simulink model "Microstick_II_33EP128MC202_Drotek_I2C_MS5611_TempAndPressure"  (Simulink 7.5)
settings: Solver=FixedStepDiscrete  StartTime=0.0  StopTime=10.0  FixedStep=0.01  RelTol=1e-3
undefined symbols (not defined in the file or in its folder): A0, A4, B10, B11, B8, B9, magnitude, Max, ms, P20, P42, P43, Pin, Resol, Slope1, Slope2, us
libraries: simulink x30, MCHP_Blockset x16
(part 1 of 2)
Description:
  | Rapid Prototyping model.
  | Require the MPLAB Blockset for Simulink v3.6 or above. [http://www.microchip.com/SimulinkBlocks]
  | Author: Lubin Kerhuel
  | 
  | Get Temperature (deg) and Pressure (Pa) from MS5611 sensor through I2C bus.
  | Apply compensation based on MS5611 datasheet and EEPROM calibration data.
  | Estimate altitude (m) from the pressure value.
  | 
  | Tested with a Microstick 2 board endowed with a dsPIC 33EP128MC202.
  | The sensor board is the IMU 10DOF V2 from Drotek [http://www.drotek.fr/shop/en/home/62-imu-10dof-mpu6050-hmc5883-ms5611.html].
  | I2C bus is connected to pin B8 (SCL) and B9 (SDA).
  | The Led connected to A0 reflect the MCU load.
settings Model: Creator=Lubin Kerhuel  LastModifiedBy=Lubin Kerhuel
settings OptimizationCC: InlineParams=on  ExpressionDepthLimit=128  OptimizeModelRefInitCode=on  LifeSpan=1
settings DebuggingCC: MultiTaskCondExecSysMsg=warning  FcnCallInpInsideContextMsg=Enable All  StateNameClashWarn=none
settings HardwareCC: ProdBitPerInt=16  ProdIntDivRoundTo=Zero  ProdEndianess=LittleEndian  ProdWordSize=16  ProdHWDeviceType=Generic->Custom
settings ModelReferenceCC: ModelReferenceNumInstancesAllowed=Single
settings RTWCC: SystemTargetFile=MCHP_dsPIC_stf.tlc  TemplateMakefile=MCHP_dsPIC.tmf  Description=Microchip Embedded Target PIC24 dsPIC30 dsPIC33 (real-time)  GenerateReport=on  ProcessScript=MCHP_dsPIC_stf_make_rtw_hook  IncludeHyperlinkInReport=on  LaunchReport=on  GenerateTraceInfo=on  GenerateTraceReport=on  GenerateTraceReportSl=on  GenerateTraceReportSf=on  GenerateTraceReportEml=on
settings CodeAppCC: IgnoreCustomStorageClasses=off  MaxIdLength=255  CustomSymbolStrType=$N$R$M_T
settings STFCustomTargetCC: TargetLibSuffix=_lib.a  IncludeMdlTerminateFcn=off  CombineOutputUpdateFcns=on  SuppressErrorStatus=on  ERTCustomFileBanners=on  SupportContinuousTime=off  SystemTargetFile=MCHP_dsPIC_stf.tlc
settings ERTTargetCC: TargetLibSuffix=_lib.a  MultiwordLength=2048  ParMdlRefBuildCompliant=off  CompOptLevelCompliant=off  IncludeMdlTerminateFcn=off  SuppressErrorStatus=on  ERTFirstTimeCompliant=off  SupportNonInlinedSFcns=on  ModelStepFunctionPrototypeControlCompliant=off  CPPClassGenCompliant=off  InlinedParameterPlacement=NonHierarchical  ERTSrcFileBannerTemplate=MCHP_dsPIC_code_template.cgt  ERTHdrFileBannerTemplate=MCHP_dsPIC_code_template.cgt  ERTDataSrcFileTemplate=MCHP_dsPIC_code_template.cgt  ERTDataHdrFileTemplate=MCHP_dsPIC_code_template.cgt  ERTCustomFileTemplate=MCHP_main.tlc  ConvertIfToSwitch=off
settings CustomProperty: DataType=string  Value=33EP128MC202
settings EnumStrPairs: String=elf

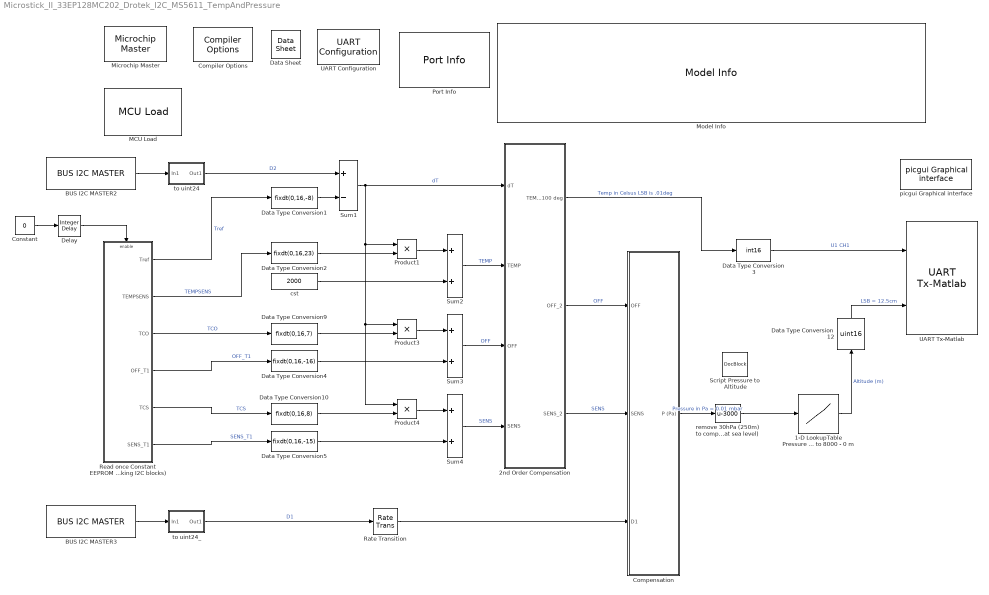
== system Microstick_II_33EP128MC202_Drotek_I2C_MS5611_TempAndPressure ==
  1-D LookupTable Pressure (Pa) to Altitude (m) Validate from 35000 to 101325 Pa  equiv to 8000 - 0 m : Lookup_n-D  NumberOfTableDimensions=1  BreakpointsForDimension1="[  35000  35358  35799  36218  36647  37086  37463  37867  38284  38639  39007  39435  39920  40363  40841  41285  41707  42156  42664  43168  43649  44137  44662  45105  45550  46088  46633  47208  47742  48308  48833  49375  49917  50484  51077  51694  52269  52806  53380  53923  54482  55078  55692  56323  56892  57456  58035  58713  59333  59883  60532  61206  61808  62536  63274  63867  64453  65183  65908  66601  67397  68144  68989  69707  70553  71274  72116  73003  73751  74585  75475  76215  77057  77852  78777  79632  80497  81475  82421  83318  84232  85034  86062  86971  87833  88819  89900  90806  91711  92745  93684  94659  95582  96686  97778  98861  99943  101077  101325]"  BreakpointsForDimension1DataTypeStr=uint32  IndexSearchMethod=Linear search  BeginIndexSearchUsingPreviousIndexResult=on  Table="floor(1e3*[  8.117494150205507  8.047307468888779  7.961635148104636  7.881024806288224  7.799269215467364  7.716406273634682  7.645877610153606  7.570932893861216  7.494252579165659  7.429504315425707  7.362891489741167  7.286054950638820  7.199797399557283  7.121747962190449  7.038306271811481  6.961505205390625  6.889127040412314  6.812766274429189  6.727161471881082  6.643042514664310  6.563500729628082  6.483523422993821  6.398277833852677  6.326975711361185  6.255920317941622  6.170761870543356  6.085312221529850  5.996031117218197  5.913901313824179  5.827657955984869  5.748390298923216  5.667276544272827  5.586880607298991  5.503529360084817  5.417163073045740  5.328158985462957  5.245984553079652  5.169899173342455  5.089261055801668  5.013621668602325  4.936395068204278  4.854760386636663  4.771404863390322  4.686513210163459  4.610620524646503  4.535998870925556  4.460007076468755  4.371798275500042  4.291854427849852  4.221500709507222  4.139153149743339  4.054386808485666  3.979312294958618  3.889311405611741  3.798936060180400  3.726933806801484  3.656311337224353  3.569058183860936  3.483182312323465  3.401808896599658  3.309182745873208  3.223060704013871  3.126556814339318  3.045306345377176  2.950436219991221  2.870307867915639  2.777558779899300  2.680796416665915  2.599934631636417  2.510555168885454  2.416062414745815  2.338179944094234  2.250303556346946  2.168043151867678  2.073183126461139  1.986300471936425  1.899166943670672  1.801559157130934  1.708043624979844  1.620171272121821  1.531418009471097  1.454180476082605  1.356035738721541  1.270039785659123  1.189159990168402  1.097429821079197  0.997804296165603  0.915051309155737  0.833054446807197  0.740167719936515  0.656538791425999  0.570418854500065  0.489551295792444  0.393651965119672  0.299663361166764  0.207285159821775  0.115806970943886  0.020789079348666  0.000124270049324])"  TableDataTypeStr=fixdt(0,16,3)  IntermediateResultsDataTypeStr=fixdt(1,32,18)  ExtrapMethod=None - Clip  UseLastTableValue=on  OutDataTypeStr=fixdt(0,16,3)  RndMeth=Simplest  FractionDataTypeStr=fixdt(1,32,18)  InputSameDT=on
  2nd Order Compensation : Subsystem
  BUS I2C MASTER2 : MCHP_Blockset/BUS I2C/BUS I2C MASTER  I2CRef=1  I2C_IntPriority=5  I2Csequence_txt="Initial-Configuration$     ---     $Start$Write Address:{[0x77]}    % Componnent address$Write Data (x1)  Write:{[0x00]}      % ADC Read$Re-Start$Read Data (x3)  Read:{D2}    % Read D2$Re-Start$Write Data (x1)  Write:{[0x48]}      % Cmd conversion D1 (OSR 4096)$Stop"  I2Csequence_num=[BFF0000000000000 40E0600000000000 412E848000000000 412E9EA0F694FA01]$[4070000000000000]$[3FF0000000000000 40E0200000000000 40F86A0000000000 40F866E066594CA2]$[4040000000000000 0000000000000000 0000000000000000 405DC00000000000]$[4050000000000000 3FF0000000000000 0000000000000000 0000000000000000]$[4008000000000000 40E0200000000000 40F86A0000000000 40F866E066594CA2]$[4060000000000000 4008000000000000]$[4008000000000000 40E0600000000000 40F86A0000000000 40F866E066594CA2]$[4050000000000000 3FF0000000000000 0000000000000000 4052000000000000]$[4000000000000000 40E0600000000000 40F86A0000000000 40F866E066594CA2]  InitialConfigurationNum=0  PIN_SDA_TXT=B9 / Pin[18]  PIN_SCL_TXT=B8 / Pin[17]  S_INPUT="[5  5]"  S_OUTPUT=[5]  S_INPUT_Size="[2  2]"  S_OUTPUT_Size=[4]  BlockingMode=off  SampleTime=[.02 0]  MCHP_MASTERLINK=Microstick_II_33EP128MC202_Drotek_I2C_MS5611_TempAndPressure/Microchip Master  MCHP_PORT={I2C 1 Clock}{SCL1}13:0:B8;{I2C 1 SDA}{SDA1}13:0:B9;  ORDERING=0
  BUS I2C MASTER3 : MCHP_Blockset/BUS I2C/BUS I2C MASTER  I2CRef=1  I2C_IntPriority=5  I2Csequence_txt="Initial-Configuration$     ---     $Start$Write Address:{[0x77]}    % Componnent address$Write Data (x1)  Write:{[0x00]}      % ADC Read$Re-Start$Read Data (x3)  Read:{D1}    % Read D1$Re-Start$Write Data (x1)  Write:{[0x58]}      % Cmd conversion D2 (OSR 4096)$Stop"  I2Csequence_num=[BFF0000000000000 40E0600000000000 412E848000000000 412E9EA0F694FA01]$[4070000000000000]$[3FF0000000000000 40E0200000000000 40F86A0000000000 40F866E066594CA2]$[4040000000000000 0000000000000000 0000000000000000 405DC00000000000]$[4050000000000000 3FF0000000000000 0000000000000000 0000000000000000]$[4008000000000000 40E0200000000000 40F86A0000000000 40F866E066594CA2]$[4060000000000000 4008000000000000]$[4008000000000000 40E0600000000000 40F86A0000000000 40F866E066594CA2]$[4050000000000000 3FF0000000000000 0000000000000000 4056000000000000]$[4000000000000000 40E0600000000000 40F86A0000000000 40F866E066594CA2]  InitialConfigurationNum=0  PIN_SDA_TXT=B9 / Pin[18]  PIN_SCL_TXT=B8 / Pin[17]  S_INPUT="[5  5]"  S_OUTPUT=[5]  S_INPUT_Size="[2  2]"  S_OUTPUT_Size=[4]  BlockingMode=off  SampleTime=[.02 0.01]  MCHP_MASTERLINK=Microstick_II_33EP128MC202_Drotek_I2C_MS5611_TempAndPressure/Microchip Master  MCHP_PORT={I2C 1 Clock}{SCL1}13:0:B8;{I2C 1 SDA}{SDA1}13:0:B9;  ORDERING=0
  Compensation : Subsystem
  Compiler Options : MCHP_Blockset/System Configuration/Compiler Options  Priority=1  LATEST_CMPLR=on  COMP_LIST=Dynamic Options  COMP_LIST_TXT=xc16 - v1.26  USE_64BIT_DOUBLE=off  MCHP_MULTITHREAD_COMPILATION=on  MCHP_MASTERLINK=Microstick_II_33EP128MC202_Drotek_I2C_MS5611_TempAndPressure/Microchip Master  OPTIMIZATION_LEVEL=3  MPLAB_LINKLIB=default  MPLAB_LINKLIB1=default  UNROLL_LOOPS=on  OMIT_FRAME_POINTER=off  PROCEDURAL_ABSTRACTION=off  MCONST=in data memory  MDATA=Use only memory below address 8192 (faster)  MSCALAR=Use only memory below address 8192 (faster)  MCODE=is less than 32768 (faster)  HEAP_SIZE=0  OMF=elf  DEBUG_INFO=off  AssemblyListing=off  ProduceHexOutput=on
  Constant : Constant  Value=0
  Data Sheet : MCHP_Blockset/System Info/Data Sheet  DOC_Type=datasheet  DOC_MCHP_Id=33FJ64MC802  DOC_FileLastCheckTime=[0 0 0 0 0 0]  cpy_MCHP_Id=33EP128MC202  MCHP_MASTERLINK=Microstick_II_33EP128MC202_Drotek_I2C_MS5611_TempAndPressure/Microchip Master
      settings: AttributesFormatString=%<cpy_MCHP_Id>
  Data Type Conversion1 : DataTypeConversion  OutDataTypeMode=Specify via dialog  OutDataType=fixdt(0,16,-8)  OutDataTypeStr=fixdt(0,16,-8)  ConvertRealWorld=Stored Integer (SI)
  Data Type Conversion10 : DataTypeConversion  OutDataTypeMode=Specify via dialog  OutDataType=fixdt(0,16,8)  OutDataTypeStr=fixdt(0,16,8)  ConvertRealWorld=Stored Integer (SI)
  Data Type Conversion12 : DataTypeConversion  OutDataTypeMode=uint16  OutDataTypeStr=uint16  ConvertRealWorld=Stored Integer (SI)
  Data Type Conversion2 : DataTypeConversion  OutDataTypeMode=Specify via dialog  OutDataType=fixdt(0,16,23)  OutDataTypeStr=fixdt(0,16,23)  ConvertRealWorld=Stored Integer (SI)
  Data Type Conversion3 : DataTypeConversion  OutDataTypeMode=int16  OutDataTypeStr=int16
  Data Type Conversion4 : DataTypeConversion  OutDataTypeMode=Specify via dialog  OutDataType=fixdt(0,16,-16)  OutDataTypeStr=fixdt(0,16,-16)  ConvertRealWorld=Stored Integer (SI)
  Data Type Conversion5 : DataTypeConversion  OutDataTypeMode=Specify via dialog  OutDataType=fixdt(0,16,-15)  OutDataTypeStr=fixdt(0,16,-15)  ConvertRealWorld=Stored Integer (SI)
  Data Type Conversion9 : DataTypeConversion  OutDataTypeMode=Specify via dialog  OutDataType=fixdt(0,16,7)  OutDataTypeStr=fixdt(0,16,7)  ConvertRealWorld=Stored Integer (SI)
  Delay : simulink/Discrete/Integer Delay  vinit=1  samptime=-1  NumDelays=1
  MCU Load : MCHP_Blockset/Profiling/MCU Load  MCULoadPin=Dynamic Options  MCULoadPin_TXT=A0 / Pin[2]  MCULoadMeasure=off  TIMER_Resolution=Dynamic Options  TIMER_Resolution_TXT="Resol: 0.1333(us)  -  Max: 8.74(ms)"  MCHP_PORT={MCU Load Pin}{MCU_Load}0:1:A0;  MCHP_TIMER_REQUEST={MCU_Load}{MCU_Load}21:5:0:0:[]:524288;  MCHP_TIMER_RESULT=[2 65535 ]  MCHP_MASTERLINK=Microstick_II_33EP128MC202_Drotek_I2C_MS5611_TempAndPressure/Microchip Master  MCHP_COMPILED_INFO="CompiledSampleTime= [Inf   0 ];CompiledInportDataTypes=[ ];CompiledInportDataWidth=[];"  Info="Timer 2:  Resol: 133.304768(ns)  -  Max: 8.73626(ms)"  SampleTime=-1
  Microchip Master : MCHP_Blockset/System Configuration/Microchip Master  Priority=1  PICREF=33EP128MC202  TIMESTEP_REF="Timer  ( 0.01s + [-9.5218e-005%] ==> 0.01s )"  BUSYFLAG=Dynamic Options  BUSYFLAG_TXT=None  PWRTEN=PWRT enabled  BOREN=Disable  BODENV=2.7V  BORV=Brown-out Reset set at 2.0V  FPWRT=64ms  DSBOREN=Deep Sleep BOR enabled in Deep Sleep  DSLPBOR=Deep Sleep BOR enabled in Deep Sleep  MCLRE=Enabled  SMCLR=MCLR pin generates a normal system Reset  PMDL1WAY=Allow only one reconfiguration  RSTPRI=Device will obtain reset instruction from Primary flash  TEMP=Not used  SOSCSRC=Analog Mode for use with crystal  SOSCSEL=Secondary oscillator configured for high-power operation  IOL1WAY=Allow only one reconfiguration  ALTVREF=Voltage reference input; ADC =RA9/RA10 Comparator =RA9;RA10  DISUVREG=Regulator is disabled  DSSWEN=Deep Sleep is controlled by the register bit DSEN  LPCFG=Disabled - regardless of RETEN  RTCBAT=RTC operation is continued through VBAT  VBTBOR=VBAT BOR enabled  WUTSEL=Default regulator start-up time used  POWERSAVE=off  FNOSC=Internal Fast RC (FRC)  FPR=ECIO w/ PLL 16x  FOSFPR=HS3 w/PLL 16x  FOS=Internal Fast RC  FRANGE=High Range  OSCILLATOR_SELECT=Internal Fast RC (FRC)  OSCILLATOR_SELECT_spd=Internal Fast RC (FRC)  QUARTZ=7.37e+06  QUARTZ_spd=7.37e+06  POSCGAIN=2x gain setting  POSCBOOST=Boost the kick start of the oscillator  SOSCGAIN=2x gain setting  SOSCBOOST=Boost the kick start of the oscillator  ACTIV_PLL=on  ACTIV_PLL_spd=on  MIPS_DESIRED=60e6  MIPS_DESIRED_spd=60e6  FPLLMUL=24x Multiplier  FPLLIDIV=12x Divider  POSCFREQ=Primary oscillator/external clock input frequency greater than 8MHz  POSCMD=XT Crystal Oscillator Mode  POSCMOD=Primary Oscillator Disabled  MIPS=60.012857142857136 * 1e6  FPLLODIV=PLL Divide by 256  PLLKEN=Clock switch to PLL source will wait until the PLL lock signal is valid.  FCKSM=Clock switching is enabled;Fail-safe Clock Monitor is disabled  FCKSMEN=Sw Disabled; Mon Disabled  IESO=Start up with FRC; then switch  DSWDTPS=1:2;147;483;648 (25.7 Days)  FWDTEN=Disable  FWDTWINSZ=Window size is 25%  FWPSA=1:512  FWPSA0=1:128  FWPSB=1:16  WDT=Disable  WDTPOST=1:32768  WDTPRE=1:128  WDTPS=1:32768  WINDIS=Watchdog Timer in Non-Window mode  WWDTEN=Non-Window mode  DSWDTEN=DSWDT enabled  DSWDTOSC=DSWDT uses Low Power RC Oscillator (LPRC)  FPBDIV=Pb_Clk is Sys_Clk/8  FSOSCEN=Enabled  LPRCSEL=High Power; High Accuracy Mode  OSCIOFCN=OSCO/CLKO/RA3 functions as CLKO (FOSC/2)  OSCIOFNC=OSC2 is general purpose digital I/O pin  LVRCFG=Low Voltage regulator is not available  PLL_96MHZ=Enabled  PLL96MHZ=96 MHz PLL Startup is enabled automatically on start-up  PLLDIV=PLL is disabled  WDTCLK=WDT uses LPRC  WDTCMX=WDT clock source is determined by the WDTCLK Configuration bits  WDTWIN=WDT Window is 25% of WDT period  APL=Aux Flash Code protect is disabled  APLK=Aux Flash Write Protection or Code Protection is Enabled  AWRP=Aux Flash may be written  BSS=No boot program Flash segment  BWP=Protection Disabled  BWRP=Boot Segment may be written  CP=Protection Disabled  EBS=No Boot EEPROM  ESS=No Segment Data EEPROM  GCP=General Segment Code protect is disabled  GSS=User program memory is not code-protected  GSS0=No protection  GSSK=General Segment Write Protection or Code Protection is Enabled  GWRP=General Segment may be written  PWP=Disable  RBS=No Boot RAM  RSS=No Secure RAM  SSS=No Secure Segment  SWRP=Secure segment may be written  WPCFG=Disable  WPDIS=Disable  WPEND=Write Protect from WPFP to the last page of memory  WPFP=Page 127 (0x1FC00)  ICESEL=Communicate on PGEC1/PGED1  ICS=Communicate on PGEC1 and PGED1  JTAGEN=Disable  COE=Reset Into Operational Mode  RES=Not used  DEBUG=Debugger is disabled  BACKBUG=Not used  BKBUG=Device resets into Operational mode  ALTI2C=I2C mapped to SDA1/SCL1 pins  ALTI2C1=I2C1 mapped to ASDA1/ASCL1 pins  ALTI2C2=I2C2 mapped to SDA2/SCL2 pins  ALTQIO=QEA1; QEB1; INDX1 are selected as inputs to QEI1  ALTSS1=SS1A is selected as the I/O pin for SPI1  CMPPOL0=Hysteresis is applied to falling edge  CMPPOL1=Hysteresis is applied to falling edge  FCANIO=Default CAN I/O  FETHIO=Default Ethernet I/O  FMIIEN=MII Enabled  FSRSSEL=SRS Priority 7  FUSBIDIO=Controlled by the USB Module  FVBUSONIO=Controlled by USB Module  HPOL=Active High  HYST0=45 mV Hysteresis  HYST1=45 mV Hysteresis  I2C1SEL=Use Default SCL1/SDA1 Pins For I2C1  LPOL=Active High  PWMPIN=Control with PORT/TRIS regs  RTCOSC=RTCC uses Secondary Oscillator (SOSC)  UPLLEN=Disabled and bypassed  UPLLIDIV=12x Divider  ATMOD8=Not used  ALTPMP=EPMP pins are in default location mode  I2C2SEL=I2C2 is multiplexed to SDA2/RA3 and SCL2/RA2  ALTADREF=AVREF+/AVREF- are mapped to RA9/RA10  ALTCVREF=CVREF+/CVREF- are mapped to RA9/RA10  PWMLOCK=PWM registers may be written without key sequence  MCHP_TIMER_REQUEST={Time Step}{TS}0:2:3:1:[]:600128.5714285714;  MCHP_TIMER_RESULT=[1 9376.0089285714239 ]  MCHP_PLLRegisters="[5    226  16387     -1]"  MCHPVAR=MCHP.fcy.periph=MCHP_Fun.Hex2num('[418C9DC9C9249248]');MCHP.fcy.MIPS=MCHP_Fun.Hex2num('[418C9DC9C9249248]');MCHP.PowerSave=0;MCHP.TimeStepFactor=MCHP_Fun.Hex2num('[3FEFFFFE00CDCD2A]');MCHP.TimeStep_Timer=1;MCHP.NTIMERS=5;MCHP.id.name='33EP128MC202';MCHP.id.N=reshape([33 128 202],1,3);MCHP.id.L=reshape({ 'EP','MC',''},1,3);MCHP.id.Arch=3;MCHP.periph.PPS.reg_RPINRx=reshape([-1 1 1 -1 -1 -1 1 -1 -1 -1 -1 -1 -1 -1 1 1 1 1 -1 -1 -1 -1 -1 -1 1 1 -1 -1 1 1 1 1 -1 -1 -1 -1 1 -1 1 -1 -1 -1 -1 -1 1 1 1 -1 -1 -1 -1 -1 1 -1 -1 -1 -1 -1 -1 -1 -1 -1 -1 -1 -1 -1 -1 -1 -1 -1 -1 -1 -1 -1 -1 1 -1 1 1 1],1,80);MCHP.PPS.dsPIC.RP=reshape([-1 -1 -1 -1 -1 -1 -1 -1 -1 -1 -1 -1 -1 -1 -1 -1 -1 -1 -1 -1 4 -1 -1 -1 -1 -1 -1 -1 -1 -1 -1 -1 -1 -1 -1 19 20 21 22 23 24 25 26 27],1,44);MCHP.PPS.dsPIC.RPI=reshape([-1 -1 -1 -1 -1 -1 -1 -1 -1 -1 -1 -1 -1 -1 -1 -1 -1 -1 -1 -1 -1 -1 -1 -1 -1 -1 -1 -1 -1 -1 -1 -1 16 17 18 -1 -1 -1 -1 -1 -1 -1 -1 -1 28 29 30 31],1,48);MCHP.PPS.dsPIC.RPINR_list=reshape({ '1','INT1','INT2','INT3','INT4','T1CK','T2CK','T3CK','T4CK','T5CK','T6CK','T7CK','T8CK','T9CK','IC1','IC2','IC3','IC4','IC5','IC6','IC7','IC8','OCFA','OCFB','FLT1','FLT2','FLT3','FLT4','QEA1','QEB1','INDX1','HOME1','QEA2','QEB2','INDX2','HOME2','U1RX','U1CTS','U2RX','U2CTS','SDI1','SCK1','SS1','44','SDI2','SCK2','SS2','48','CSDIR','CSCK','COFS','52','C1RX','C2RX','U3RX','U3CTS','U4RX','U4CTS','SDI3','SCK3','SS3','62','SDI4','SCK4','SS4','66','IC9','IC10','IC11','IC12','IC13','IC14','IC15','IC16','OCFC','SYNCI1','SYNCI2','DTCMP1','DTCMP2','DTCMP3','DTCMP4','DTCMP5','DTCMP6','DTCMP7','FLT5','FLT6','FLT7','FLT8','89','SENT1','SENT2','92'},1,92);MCHP.PPS.dsPIC.RPOR_list=reshape({ '1','U1TX','U1RTS','U2TX','U2RTS','SDO1','SCK1','SS1','SDO2','SCK2','SS2','CSDO','CSCK','COFS','C1TX','C2TX','OC1','OC2','OC3','OC4','OC5','OC6','OC7','OC8','C1OUT','C2OUT','C3OUT','U3TX','U3RTS','U4TX','U4RTS','SDO3','SCK3','SS3','SDO4','SCK4','SS4','OC9','OC10','OC11','OC12','OC13','OC14','OC15','OC16','SYNCO1','SYNCO2','QEI1CCMP','QEI2CCMP','REFCLK','C4OUT','C5OUT','52','53','54','55','56','SENT1','SENT2'},1,59);MCHP.PPS.map_RPnR_RPORx=reshape([20 35 36 37 38 39 40 41 42 43],1,10);MCHP.Rx=reshape([2 4 -1 -1 -1 -1 -1 -1 -1 -1 -1 3 5 -1 -1 -1 -1 -1 -1 -1 -1 -1 9 6 -1 -1 -1 -1 -1 -1 -1 -1 -1 10 7 -1 -1 -1 -1 -1 -1 -1 -1 -1 12 11 -1 -1 -1 -1 -1 -1 -1 -1 -1 -1 14 -1 -1 -1 -1 -1 -1 -1 -1 -1 -1 15 -1 -1 -1 -1 -1 -1 -1 -1 -1 -1 16 -1 -1 -1 -1 -1 -1 -1 -1 -1 -1 17 -1 -1 -1 -1 -1 -1 -1 -1 -1 -1 18 -1 -1 -1 -1 -1 -1 -1 -1 -1 -1 21 -1 -1 -1 -1 -1 -1 -1 -1 -1 -1 22 -1 -1 -1 -1 -1 -1 -1 -1 -1 -1 23 -1 -1 -1 -1 -1 -1 -1 -1 -1 -1 24 -1 -1 -1 -1 -1 -1 -1 -1 -1 -1 25 -1 -1 -1 -1 -1 -1 -1 -1 -1 -1 26 -1 -1 -1 -1 -1 -1 -1 -1 -1],11,16);MCHP.ADC.ANtype=reshape([3 0],1,2);MCHP.ADC.ADCONx=reshape([47103 59391 40959 263 0 0],1,6);MCHP.ADC.ADCHS_0=reshape([40863 1799],1,2);MCHP.ADC.Flags=reshape([1 0],1,2);MCHP.ADC.Buffer=reshape([16 -1],1,2);MCHP.ADC.port=reshape([0 1 16 17 18 19 -1 -1 -1 -1 -1 -1 -1 -1 -1 -1 -1 -1 -1 -1 -1 -1 -1 -1 -1 -1 -1 -1 -1 -1 -1 -1 -1 -1 -1 -1 -1 -1 -1 -1 -1 -1 -1 -1 -1 -1 -1 -1 -1 -1 -1 -1 -1 -1 -1 -1 -1],1,57);MCHP.ADC.port_VrefP=17;MCHP.ADC.port_VrefM=16;MCHP.ADC.port_AVdd=-1;MCHP.ADC.port_AVss=-1;MCHP.memory.RAM=16384;MCHP.memory.RAM_XBegin=4096;MCHP.memory.RAM_YBegin=12288;MCHP.memory.RAM_dma=reshape([-1 -1],1,2);MCHP.DMA.Num=4;MCHP.DMA.CNTmax=16383;MCHP.QEI.QEICONx=reshape([49023 -1 -1 -1 -1 -1],1,6);MCHP.QEI.QEItype=1;MCHP.QEI.Port_QEI_INDX=reshape([-1 -1],1,2);MCHP.QEI.Port_QEI_QEA=reshape([-1 -1],1,2);MCHP.QEI.Port_QEI_QEB=reshape([-1 -1],1,2);MCHP.QEI.Port_QEI_UPDN=reshape([-1 -1],1,2);MCHP.INT.Port=reshape([23 32767 32767 -1 -1],1,5);MCHP.PWM_HS.Flags=reshape([3 1 0],1,3);MCHP.PWM.port_FLT=reshape([-1 -1 -1 -1 -1 -1 -1 -1 -1 -1 -1 -1 -1 -1 -1 -1 -1 -1 -1 -1 -1 -1 -1 -1 -1 -1 -1 -1 -1 -1 -1 -1 20],1,33);MCHP.PWM.PWMRef=-1;MCHP.PWM.Flag=0;MCHP.PWM.Port_PWM_l=reshape([31 -1 29 -1 27 -1 -1 -1 -1 -1 -1 -1 -1 -1 -1 -1 -1 -1],2,9);MCHP.PWM.Port_PWM_h=reshape([30 -1 28 -1 26 -1 -1 -1 -1 -1 -1 -1 -1 -1 -1 -1 -1 -1],2,9);MCHP.IC.Port=reshape([32767 32767 32767 32767 0 0 0 0 0 0 0 0 0 0 0 0],1,16);MCHP.IC.type=1;MCHP.OC.Port=reshape([32767 32767 32767 32767 0 0 0 0 0 0 0 0 0 0 0 0],1,16);MCHP.OC.type=1;MCHP.CN.Port=reshape([-1 -1 -1 -1 -1 -1 -1 -1 -1 -1 -1 -1 -1 -1 -1 -1 -1 -1 -1 -1 -1 -1 -1 -1 -1 -1 -1 -1 -1 -1 -1 -1 -1 -1 -1 -1 -1 -1 -1 -1 -1 -1 -1 -1 -1 -1 -1 -1 -1 -1 -1 -1 -1 -1 -1 -1 -1 -1 -1 -1 -1 -1 -1 -1 -1 -1 -1 -1 -1 -1 -1 -1 -1 -1 -1 -1 -1 -1 -1 -1 -1 -1 -1 -1 -1],1,85);MCHP.CN.PullUp=reshape([31 65535 0 0 0 0 0 0 0 0 0],1,11);MCHP.CN.type=1;MCHP.CN.Flag_PullDown=1;MCHP.SPI.Refs=reshape([1 2 0 0 0 0],1,6);MCHP.SPI.SPIxCON1=8191;MCHP.SPI.SPIxCON2=57347;MCHP.SPI.Port_SDI=reshape([25 -1 -1 -1 -1 -1],1,6);MCHP.SPI.Port_SDO=reshape([24 -1 -1 -1 -1 -1],1,6);MCHP.SPI.Port_SCK=reshape([23 -1 -1 -1 -1 -1],1,6);MCHP.SPI.Port_SS=reshape([16 -1 -1 -1 -1 -1],1,6);MCHP.I2C.Refs=reshape([1 2 0 0 0],1,5);MCHP.I2C.I2CxCON=49151;MCHP.I2C.NewRegName=1;MCHP.I2C.Port_SDA=reshape([-1 -1 -1 -1 -1],1,5);MCHP.I2C.Port_SCL=reshape([-1 -1 -1 -1 -1],1,5);MCHP.I2C.Port_ASDA=reshape([25 21 -1 -1 -1],1,5);MCHP.I2C.Port_ASCL=reshape([24 22 -1 -1 -1],1,5);MCHP.I2C.Fuse_Port_SCL_SDA=reshape([3 1 4 1 -1 -1 -1 -1 -1 -1],2,5);MCHP.I2C.Fuse_Port_ASCL_ASDA=reshape([3 2 4 2 -1 -1 -1 -1 -1 -1],2,5);MCHP.Comp.Port_CVrefin=-1;MCHP.Comp.Port_CVref=-1;MCHP.Comp.Port_CVref1O=24;MCHP.Comp.Port_CVref2O=4;MCHP.Comp.Port_CxOUT=reshape([32767 32767 32767 32767 -1],1,5);MCHP.Comp.Port_OAxOUT=reshape([17 0 -1 -1 -1],1,5);MCHP.Comp.Port_CxINP=reshape([18 1 -1 -1 -1],1,5);MCHP.Comp.Port_CxINM=reshape([19 -1 -1 -1 16 -1 -1 -1 -1 -1 -1 -1 -1 -1 -1 -1 -1 -1 -1 -1],4,5);MCHP.Comp.nComp=reshape([4 0 0],1,3);MCHP.Comp.OpAmp=3;MCHP.Comp.CVRCON=reshape([17663 0],1,2);MCHP.UART.port_Rx=reshape([32767 32767 -1 -1 -1 -1],1,6);MCHP.UART.port_Tx=reshape([32767 32767 -1 -1 -1 -1],1,6);MCHP.UART.port_ARx=reshape([-1 -1],1,2);MCHP.UART.port_ATx=reshape([-1 -1],1,2);MCHP.UART.port_RTS=reshape([32767 32767 -1 -1 -1 -1],1,6);MCHP.UART.port_CTS=reshape([32767 32767 -1 -1 -1 -1],1,6);MCHP.UART.reg_UxMODE=reshape([48127 48127 -1 -1 -1 -1],1,6);MCHP.UART.reg_UxSTA=reshape([61439 61439 -1 -1 -1 -1],1,6);  MCHP_CRC=2807621  BTMODE=Device is in Single Boot (legacy) mode  RES1=Not used  PLLSS=PLL is fed by the Primary oscillator  RES2=Not used  ALTCMPI=C1INC is on RB13; C2INC is on RB9 and C3INC is on RA0  BOREN1=BOR Enabled [When BOREN=1]  ALTRB6=Append the RP6/ASCL1/PMPD6 functions of RB6 to RA1 pin functions  RETCFG=Retention regulator is not available  DFMCY=Not used  BSS2=No Boot Segment  BSEN=No Boot Segment  CWRP=Configuration Segment may be written  CSS=No Protection (other than CWRP)  AIVTDIS=Disable Alternate Vector Table  BSLIM=Not used  WDTEN=Disable  BTSWP=Not used  DBCC=Not used  CTXT1=Not Assigned  CTXT2=Not Assigned  SEQNUM=Not used  nSEQNUM=Not used  BOREN0=Enabled  DMTIVT=Not used  DMTCNT=2^31 (2147483648)  DMTEN=Dead Man Timer is Enabled and cannot be disabled by software  ON=Not used  USERID=Not used  RESERVED1=Not used  PGL1WAY=Allow only one reconfiguration  FPLLRNG=34-68 MHz Input  FPLLICLK=FRC is input to the System PLL  FPLLMULT=PLL Multiply by 128  UPLLFSEL=USB PLL input is 24 MHz  DMTINTV=Window/Interval value is 127/128 counter value  WDTSPGM=WDT stops during Flash programming  FDMTEN=Deadman Timer is disabled  TRCEN=Trace features in the CPU are enabled  BOOTISA=Boot code and Exception code is MIPS32  FECCCON=ECC and Dynamic ECC are disabled (ECCCON bits are writable)  EXTDDRSIZE=External DDR2 Size is 128 MB  FSLEEP=Flash is powered down when the device is in Sleep mode  DBGPER=Allow CPU access to all permission regions  EJTAGBEN=Normal EJTAG functionality  TSEQ=Not used  CSEQ=Not used
  Model Info : simulink/Model-Wide Utilities/Model Info  SystemSampleTime=-1  InitialBlockCM=none  BlockCM=none  Frame=off  DisplayStringWithTags=%<Description>  HorizontalTextAlignment=Center  LeftAlignmentValue=0.5  SourceBlockDiagram=Microstick_II_33EP128MC202_Drotek_I2C_MS5611_TempAndPressure  TagMaxNumber=20
  Port Info : MCHP_Blockset/System Info/Port Info  MCHP_MASTERLINK=Microstick_II_33EP128MC202_Drotek_I2C_MS5611_TempAndPressure/Microchip Master
  Product1 : Product
  Product3 : Product
  Product4 : Product
  Rate Transition : RateTransition  Integrity=off  Deterministic=off
  Read once Constant EEPROM Calibration data From MS5611 (Blocking I2C blocks) : Subsystem
  Script Pressure to Altitude : simulink/Model-Wide Utilities/DocBlock  SystemSampleTime=-1  DocumentType=Text
      content=|
      | %% The script to compute the lookup table to translate pressure from Pascal unit (Pa) to meters (m) here after
      |
      | func = '44331.5-4946.62*x.^0.190263';   % Model from Pressure (Pa) to altitude (m)
      |
      | xmin = 35000;  xmax = 101325; % Min and max pressure
      | xdt = ufix(32); xscale = 1; % x scaling
      |
      | ydt = ufix(16);
      | yscale = 2^-3;  % y output is altitude, in m. Max value is 8000 thus 13 bits are required for integer part and 3 can be used as fractional part.
      | % y LSB is 12.5 cm
      |
      | rndmeth = 'Floor';
      | errmax = [.2];
      | nptsmax = 256;
      | %spacing = 'even';
      |
      | % Compute lookup table (might take few seconds to compute)
      | [xdata,ydata,errworst] = fixpt_look1_func_approx(func,xmin,xmax,xdt,xscale,ydt,yscale,rndmeth,errmax,nptsmax);
      | % Check results
      | fixpt_look1_func_plot(xdata,ydata,func,xmin,xmax,xdt,xscale,ydt,yscale,rndmeth);
  Sum1 : Sum  Inputs=+-  AccumDataTypeStr=fixdt(1,24,0)  OutDataTypeStr=Inherit: Same as accumulator
  Sum2 : Sum  OutMin=-4000  OutMax=8500  OutDataTypeMode=Specify via dialog  OutDataType=fixdt(1,32,17)  OutDataTypeStr=fixdt(1,32,17)
  Sum3 : Sum  OutMin=-8589672450  OutMax=12884705280  OutDataTypeMode=Specify via dialog  OutDataType=fixdt(1,41,6)  OutDataTypeStr=fixdt(1,41,6)
  Sum4 : Sum  OutMin=-4294836225  OutMax=6442352640  OutDataTypeMode=Specify via dialog  OutDataType=fixdt(1,41,7)  OutDataTypeStr=fixdt(1,41,7)
  UART Configuration : MCHP_Blockset/BUS UART/UART Configuration  UART_REF=1  BAUD_Choice=Dynamic Options  BAUD_Choice_TXT="115200         [+0.18%]"  BAUD_Choice_IR=Dynamic Options  BAUD_Choice_IR_TXT=[]  BAUD_Custom=115200  IRDA=off  ALT_IO=on  PIN_RX=Dynamic Options  PIN_RX_TXT=B11 / P43 / Pin[22]  PIN_TX=Dynamic Options  PIN_TX_TXT=B10 / P42 / Pin[21]  FlowControl=None  PIN_CTS=Dynamic Options  PIN_CTS_TXT=A4 / P20 / Pin[12]  PIN_RTS=Dynamic Options  PIN_RTS_TXT=A4 / P20 / Pin[12]  MCHP_PORT="{UART1  Tx}{U1TX}3:1:P42;"  MCHP_MASTERLINK=Microstick_II_33EP128MC202_Drotek_I2C_MS5611_TempAndPressure/Microchip Master  MCHP_COM_ExtPil=off  TX_IMPLEMENTATION=Circular Buffer  TX_INT_PRIORITY=5  TX_INT_WHEN=is empty & last char is sent  TX_CIRCULAR_SIZE=32  TX_DMA_CHANNEL="0   (Lowest Priority)"  TX_DMA_SIZE=[]  RX_IMPLEMENTATION=Do not implement Rx  RX_INT_PRIORITY=1  RX_INT_WHEN=receive 1 character  RX_CIRCULAR_SIZE=32  InitSequence_chkbox=off  BAUD_Choice_InitSeq=Dynamic Options  BAUD_Choice_InitSeq_TXT=0  BAUD_Choice_IR_InitSeq=Dynamic Options  BAUD_Choice_IR_InitSeq_TXT=0  BAUD_Custom_InitSeq=0  InitSequence='Hello World'
  UART Tx-Matlab : MCHP_Blockset/BUS UART/UART Tx-Matlab  UART_REF=1  CHANNELS=[1:2]  AllOrNothing=off  SampleTime=-1  MCHP_MASTERLINK=Microstick_II_33EP128MC202_Drotek_I2C_MS5611_TempAndPressure/Microchip Master  MCHP_COMPILED_INFO="CompiledSampleTime= [0.02   0 ];CompiledInportDataTypes=[  4   5 ];CompiledInportDataWidth=[1  1];"
  cst : Constant  Value=2000  OutDataTypeMode=uint16  OutDataTypeStr=uint16
  picgui Graphical interface : MCHP_Blockset/BUS UART/picgui Graphical interface  Nothing=0
  remove 30hPa (250m) to compensate for bad weather forecast (avoir neg value at sea level) : Bias  Bias=-3000
  to uint24 : Subsystem
  to uint24_ : Subsystem
  wires:
  BUS I2C MASTER2/1 -> to uint24/1(In1)
  to uint24/1(Out1) -> Sum1/1  "D2"
  Data Type Conversion1/1 -> Sum1/2
  Sum1/1 -> Product3/1, Product4/1, Product1/1, 2nd Order Compensation/1(dT)  "dT"
  Product1/1 -> Sum2/1
  Data Type Conversion2/1 -> Product1/2
  Product3/1 -> Sum3/1
  Data Type Conversion4/1 -> Sum3/2
  Product4/1 -> Sum4/1
  Data Type Conversion5/1 -> Sum4/2
  Data Type Conversion9/1 -> Product3/2
  Data Type Conversion10/1 -> Product4/2
  Delay/1 -> Read once Constant EEPROM Calibration data From MS5611 (Blocking I2C blocks)/Enable
  Constant/1 -> Delay/1
  cst/1 -> Sum2/2
  Sum2/1 -> 2nd Order Compensation/2(TEMP)  "TEMP"
  Sum3/1 -> 2nd Order Compensation/3(OFF)  "OFF"
  Sum4/1 -> 2nd Order Compensation/4(SENS)  "SENS"
  to uint24_/1(Out1) -> Rate Transition/1  "D1"
  2nd Order Compensation/3(SENS_2) -> Compensation/2(SENS)  "SENS"
  2nd Order Compensation/2(OFF_2) -> Compensation/1(OFF)  "OFF"
  Rate Transition/1 -> Compensation/3(D1)
  BUS I2C MASTER3/1 -> to uint24_/1(In1)
  Read once Constant EEPROM Calibration data From MS5611 (Blocking I2C blocks)/1(Tref) -> Data Type Conversion1/1  "Tref"
  Read once Constant EEPROM Calibration data From MS5611 (Blocking I2C blocks)/2(TEMPSENS) -> Data Type Conversion2/1  "TEMPSENS"
  Read once Constant EEPROM Calibration data From MS5611 (Blocking I2C blocks)/3(TCO) -> Data Type Conversion9/1  "TCO"
  Read once Constant EEPROM Calibration data From MS5611 (Blocking I2C blocks)/4(OFF_T1) -> Data Type Conversion4/1  "OFF_T1"
  Read once Constant EEPROM Calibration data From MS5611 (Blocking I2C blocks)/5(TCS) -> Data Type Conversion10/1  "TCS"
  Read once Constant EEPROM Calibration data From MS5611 (Blocking I2C blocks)/6(SENS_T1) -> Data Type Conversion5/1  "SENS_T1"
  2nd Order Compensation/1(TEMP 1/100 deg) -> Data Type Conversion3/1  "Temp in Celsus LSB is .01deg"
  Data Type Conversion3/1 -> UART Tx-Matlab/1  "U1 CH1"
  Compensation/1(P (Pa)) -> remove 30hPa (250m) to compensate for bad weather forecast (avoir neg value at sea level)/1  "Pressure in Pa = 0.01 mbar"
  remove 30hPa (250m) to compensate for bad weather forecast (avoir neg value at sea level)/1 -> 1-D LookupTable Pressure (Pa) to Altitude (m) Validate from 35000 to 101325 Pa  equiv to 8000 - 0 m/1
  1-D LookupTable Pressure (Pa) to Altitude (m) Validate from 35000 to 101325 Pa  equiv to 8000 - 0 m/1 -> Data Type Conversion12/1  "Altitude (m)"
  Data Type Conversion12/1 -> UART Tx-Matlab/2  "LSB = 12.5cm"

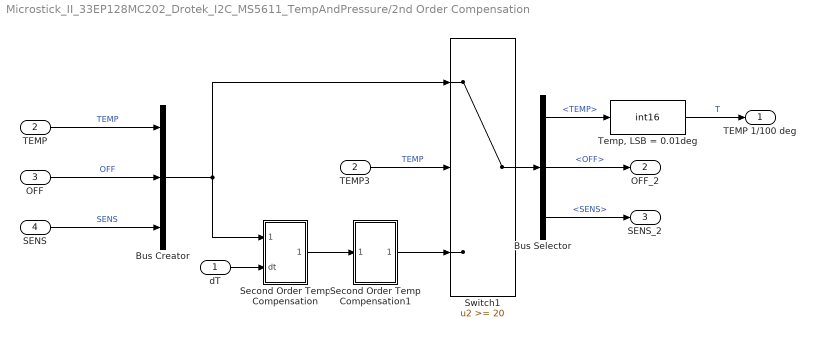
== system Microstick_II_33EP128MC202_Drotek_I2C_MS5611_TempAndPressure/2nd Order Compensation ==
  dT : Inport
  TEMP : Inport  Port=2
  OFF : Inport  Port=3
  SENS : Inport  Port=4
  Bus Creator : BusCreator  Inputs=3
  Bus Selector : BusSelector  OutputSignals=TEMP,OFF,SENS
  Second Order Temp Compensation : Subsystem
  Second Order Temp Compensation1 : Subsystem
  Switch1 : Switch  Threshold=20  InputSameDT=on
  TEMP3 : InportShadow  Port=2
  "Temp, LSB = 0.01deg" : DataTypeConversion  OutDataTypeMode=int16  OutDataTypeStr=int16
  TEMP 1/100 deg : Outport
  OFF_2 : Outport  Port=2
  SENS_2 : Outport  Port=3
  wires:
  TEMP3/1 -> Switch1/2  "TEMP"
  Switch1/1 -> Bus Selector/1
  TEMP/1 -> Bus Creator/1  "TEMP"
  OFF/1 -> Bus Creator/2  "OFF"
  SENS/1 -> Bus Creator/3  "SENS"
  Bus Creator/1 -> Switch1/1, Second Order Temp Compensation/1(In3)
  Second Order Temp Compensation/1(Out1) -> Second Order Temp Compensation1/1(In3)
  Second Order Temp Compensation1/1(Out1) -> Switch1/3
  Bus Selector/1 -> "Temp, LSB = 0.01deg"/1  "<TEMP>"
  Bus Selector/2 -> OFF_2/1  "<OFF>"
  Bus Selector/3 -> SENS_2/1  "<SENS>"
  dT/1 -> Second Order Temp Compensation/2(dt)
  "Temp, LSB = 0.01deg"/1 -> TEMP 1/100 deg/1  "T"

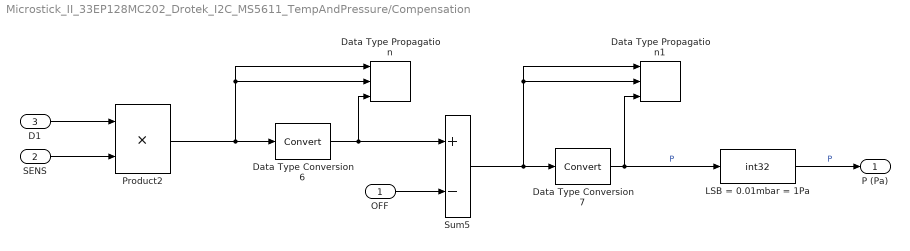
== system Microstick_II_33EP128MC202_Drotek_I2C_MS5611_TempAndPressure/Compensation ==
  OFF : Inport
  SENS : Inport  Port=2
  D1 : Inport  Port=3
  Data Type Propagation : simulink/Signal Attributes/Data Type Propagation  PropDataType=fixdt(1, 16)  IfRefDouble=double  IfRefSingle=single  IsSigned=IsSigned1 or IsSigned2  NumBitsBase=NumBits1  NumBitsMult=1  NumBitsAdd=0  NumBitsAllowFinal=1:128  PropScaling=2^-10  ValuesUsedBestPrec=[5 -7]  SlopeBase=min([Slope1 Slope2])  SlopeMult=2^-21  SlopeAdd=0  BiasBase=Bias1  BiasMult=1  BiasAdd=0
  Data Type Propagation1 : simulink/Signal Attributes/Data Type Propagation  PropDataType=fixdt(1, 16)  IfRefDouble=double  IfRefSingle=single  IsSigned=IsSigned1 or IsSigned2  NumBitsBase=NumBits1  NumBitsMult=1  NumBitsAdd=0  NumBitsAllowFinal=1:128  PropScaling=2^-10  ValuesUsedBestPrec=[5 -7]  SlopeBase=min([Slope1 Slope2])  SlopeMult=2^-15  SlopeAdd=0  BiasBase=Bias1  BiasMult=1  BiasAdd=0
  Data Type Conversion6 : DataTypeConversion  ConvertRealWorld=Stored Integer (SI)
  Data Type Conversion7 : DataTypeConversion  ConvertRealWorld=Stored Integer (SI)
  LSB = 0.01mbar = 1Pa : DataTypeConversion  OutDataTypeMode=int32  OutDataTypeStr=int32
  Product2 : Product  OutMin=-4294836225*(2^24-1)  OutMax=6442352640*(2^24-1)  OutDataTypeMode=Specify via dialog  OutDataType=fixdt(1,64,6)  OutDataTypeStr=fixdt(1,64,6)
  Sum5 : Sum  Inputs=+-  OutDataTypeStr=Inherit: Same as accumulator
  P (Pa) : Outport
  wires:
  Data Type Conversion7/1 -> LSB = 0.01mbar = 1Pa/1, Data Type Propagation1/3  "P"
  D1/1 -> Product2/1
  SENS/1 -> Product2/2
  Product2/1 -> Data Type Propagation/1, Data Type Propagation/2, Data Type Conversion6/1
  Data Type Conversion6/1 -> Data Type Propagation/3, Sum5/1
  OFF/1 -> Sum5/2
  Sum5/1 -> Data Type Propagation1/2, Data Type Propagation1/1, Data Type Conversion7/1
  LSB = 0.01mbar = 1Pa/1 -> P (Pa)/1  "P"

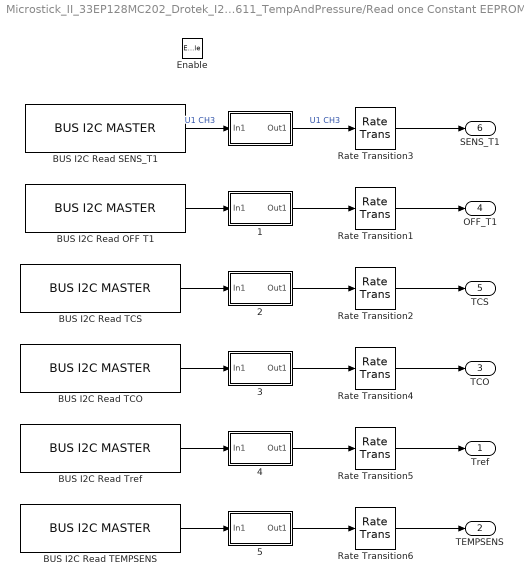
== system Microstick_II_33EP128MC202_Drotek_I2C_MS5611_TempAndPressure/Read once Constant EEPROM Calibration data From MS5611 (Blocking I2C blocks) ==
  Enable : EnablePort
  " " : Subsystem
  " 1" : Subsystem
  " 2" : Subsystem
  " 3" : Subsystem
  " 4" : Subsystem
  " 5" : Subsystem
  BUS I2C Read OFF T1 : MCHP_Blockset/BUS I2C/BUS I2C MASTER  I2CRef=1  I2C_IntPriority=5  I2Csequence_txt="Initial-Configuration$     ---     $Start$Write Address:{[0x77]}    % Componnent address$Write Data (x1)  Write:{[0xA4]}      % PROM Read$Re-Start$Read Data (x2)  Read:{OFF_T1}    % Read OFF_T1$Stop"  I2Csequence_num=[BFF0000000000000 40E0600000000000 412E848000000000 412E9EA0F694FA01]$[4070000000000000]$[3FF0000000000000 40E0200000000000 40F86A0000000000 40F866E066594CA2]$[4040000000000000 0000000000000000 0000000000000000 405DC00000000000]$[4050000000000000 3FF0000000000000 0000000000000000 4064800000000000]$[4008000000000000 40E0200000000000 40F86A0000000000 40F866E066594CA2]$[4060000000000000 4000000000000000]$[4000000000000000 40E0600000000000 40F86A0000000000 410065D9C7810E65]  InitialConfigurationNum=0  PIN_SDA_TXT=B9 / Pin[18]  PIN_SCL_TXT=B8 / Pin[17]  S_INPUT="[5  5]"  S_OUTPUT=[5]  S_INPUT_Size="[2  2]"  S_OUTPUT_Size=[4]  BlockingMode=on  SampleTime=-1  MCHP_MASTERLINK=Microstick_II_33EP128MC202_Drotek_I2C_MS5611_TempAndPressure/Microchip Master  MCHP_PORT={I2C 1 Clock}{SCL1}13:0:B8;{I2C 1 SDA}{SDA1}13:0:B9;  ORDERING=0
  BUS I2C Read SENS_T1 : MCHP_Blockset/BUS I2C/BUS I2C MASTER  I2CRef=1  I2C_IntPriority=5  I2Csequence_txt="Initial-Configuration$     ---     $Start$Write Address:{[0x77]}    % Componnent address$Write Data (x1)  Write:{[0xA2]}      % PROM Read$Re-Start$Read Data (x2)  Read:{SENS_T1}    % Read SENS_T1$Stop"  I2Csequence_num=[BFF0000000000000 40E0600000000000 412E848000000000 412E9EA0F694FA01]$[4070000000000000]$[3FF0000000000000 40E0200000000000 40F86A0000000000 40F866E066594CA2]$[4040000000000000 0000000000000000 0000000000000000 405DC00000000000]$[4050000000000000 3FF0000000000000 0000000000000000 4064400000000000]$[4008000000000000 40E0200000000000 40F86A0000000000 40F866E066594CA2]$[4060000000000000 4000000000000000]$[4000000000000000 40E0600000000000 40F86A0000000000 410065D9C7810E65]  InitialConfigurationNum=0  PIN_SDA_TXT=B9 / Pin[18]  PIN_SCL_TXT=B8 / Pin[17]  S_INPUT="[5  5]"  S_OUTPUT=[5]  S_INPUT_Size="[2  2]"  S_OUTPUT_Size=[4]  BlockingMode=on  SampleTime=-1  MCHP_MASTERLINK=Microstick_II_33EP128MC202_Drotek_I2C_MS5611_TempAndPressure/Microchip Master  MCHP_PORT={I2C 1 Clock}{SCL1}13:0:B8;{I2C 1 SDA}{SDA1}13:0:B9;  ORDERING=0
  BUS I2C Read TCO : MCHP_Blockset/BUS I2C/BUS I2C MASTER  I2CRef=1  I2C_IntPriority=5  I2Csequence_txt="Initial-Configuration$     ---     $Start$Write Address:{[0x77]}    % Componnent address$Write Data (x1)  Write:{[0xA8]}      % PROM Read$Re-Start$Read Data (x2)  Read:{TCO}    % Read TCO$Stop"  I2Csequence_num=[BFF0000000000000 40E0600000000000 412E848000000000 412E9EA0F694FA01]$[4070000000000000]$[3FF0000000000000 40E0200000000000 40F86A0000000000 40F866E066594CA2]$[4040000000000000 0000000000000000 0000000000000000 405DC00000000000]$[4050000000000000 3FF0000000000000 0000000000000000 4065000000000000]$[4008000000000000 40E0200000000000 40F86A0000000000 40F866E066594CA2]$[4060000000000000 4000000000000000]$[4000000000000000 40E0600000000000 40F86A0000000000 410065D9C7810E65]  InitialConfigurationNum=0  PIN_SDA_TXT=B9 / Pin[18]  PIN_SCL_TXT=B8 / Pin[17]  S_INPUT="[5  5]"  S_OUTPUT=[5]  S_INPUT_Size="[2  2]"  S_OUTPUT_Size=[4]  BlockingMode=on  SampleTime=-1  MCHP_MASTERLINK=Microstick_II_33EP128MC202_Drotek_I2C_MS5611_TempAndPressure/Microchip Master  MCHP_PORT={I2C 1 Clock}{SCL1}13:0:B8;{I2C 1 SDA}{SDA1}13:0:B9;  ORDERING=0
  BUS I2C Read TCS : MCHP_Blockset/BUS I2C/BUS I2C MASTER  I2CRef=1  I2C_IntPriority=5  I2Csequence_txt="Initial-Configuration$     ---     $Start$Write Address:{[0x77]}    % Componnent address$Write Data (x1)  Write:{[0xA6]}      % PROM Read$Re-Start$Read Data (x2)  Read:{TCS}    % Read TCS$Stop"  I2Csequence_num=[BFF0000000000000 40E0600000000000 412E848000000000 412E9EA0F694FA01]$[4070000000000000]$[3FF0000000000000 40E0200000000000 40F86A0000000000 40F866E066594CA2]$[4040000000000000 0000000000000000 0000000000000000 405DC00000000000]$[4050000000000000 3FF0000000000000 0000000000000000 4064C00000000000]$[4008000000000000 40E0200000000000 40F86A0000000000 40F866E066594CA2]$[4060000000000000 4000000000000000]$[4000000000000000 40E0600000000000 40F86A0000000000 410065D9C7810E65]  InitialConfigurationNum=0  PIN_SDA_TXT=B9 / Pin[18]  PIN_SCL_TXT=B8 / Pin[17]  S_INPUT="[5  5]"  S_OUTPUT=[5]  S_INPUT_Size="[2  2]"  S_OUTPUT_Size=[4]  BlockingMode=on  SampleTime=-1  MCHP_MASTERLINK=Microstick_II_33EP128MC202_Drotek_I2C_MS5611_TempAndPressure/Microchip Master  MCHP_PORT={I2C 1 Clock}{SCL1}13:0:B8;{I2C 1 SDA}{SDA1}13:0:B9;  ORDERING=0
  BUS I2C Read TEMPSENS : MCHP_Blockset/BUS I2C/BUS I2C MASTER  I2CRef=1  I2C_IntPriority=5  I2Csequence_txt="Initial-Configuration$     ---     $Start$Write Address:{[0x77]}    % Componnent address$Write Data (x1)  Write:{[0xAC]}      % PROM Read$Re-Start$Read Data (x2)  Read:{TEMPSENS}    % Read TEMPSENS$Stop"  I2Csequence_num=[BFF0000000000000 40E0600000000000 412E848000000000 412E9EA0F694FA01]$[4070000000000000]$[3FF0000000000000 40E0200000000000 40F86A0000000000 40F866E066594CA2]$[4040000000000000 0000000000000000 0000000000000000 405DC00000000000]$[4050000000000000 3FF0000000000000 0000000000000000 4065800000000000]$[4008000000000000 40E0200000000000 40F86A0000000000 40F866E066594CA2]$[4060000000000000 4000000000000000]$[4000000000000000 40E0600000000000 40F86A0000000000 410065D9C7810E65]  InitialConfigurationNum=0  PIN_SDA_TXT=B9 / Pin[18]  PIN_SCL_TXT=B8 / Pin[17]  S_INPUT="[5  5]"  S_OUTPUT=[5]  S_INPUT_Size="[2  2]"  S_OUTPUT_Size=[4]  BlockingMode=on  SampleTime=-1  MCHP_MASTERLINK=Microstick_II_33EP128MC202_Drotek_I2C_MS5611_TempAndPressure/Microchip Master  MCHP_PORT={I2C 1 Clock}{SCL1}13:0:B8;{I2C 1 SDA}{SDA1}13:0:B9;  ORDERING=0
  BUS I2C Read Tref : MCHP_Blockset/BUS I2C/BUS I2C MASTER  I2CRef=1  I2C_IntPriority=5  I2Csequence_txt="Initial-Configuration$     ---     $Start$Write Address:{[0x77]}    % Componnent address$Write Data (x1)  Write:{[0xAA]}      % PROM Read$Re-Start$Read Data (x2)  Read:{Tref}    % Read Tref$Stop"  I2Csequence_num=[BFF0000000000000 40E0600000000000 412E848000000000 412E9EA0F694FA01]$[4070000000000000]$[3FF0000000000000 40E0200000000000 40F86A0000000000 40F866E066594CA2]$[4040000000000000 0000000000000000 0000000000000000 405DC00000000000]$[4050000000000000 3FF0000000000000 0000000000000000 4065400000000000]$[4008000000000000 40E0200000000000 40F86A0000000000 40F866E066594CA2]$[4060000000000000 4000000000000000]$[4000000000000000 40E0600000000000 40F86A0000000000 410065D9C7810E65]  InitialConfigurationNum=0  PIN_SDA_TXT=B9 / Pin[18]  PIN_SCL_TXT=B8 / Pin[17]  S_INPUT="[5  5]"  S_OUTPUT=[5]  S_INPUT_Size="[2  2]"  S_OUTPUT_Size=[4]  BlockingMode=on  SampleTime=-1  MCHP_MASTERLINK=Microstick_II_33EP128MC202_Drotek_I2C_MS5611_TempAndPressure/Microchip Master  MCHP_PORT={I2C 1 Clock}{SCL1}13:0:B8;{I2C 1 SDA}{SDA1}13:0:B9;  ORDERING=0
  Rate Transition{1..6} (6 alike) : RateTransition  Integrity=off  Deterministic=off
  Tref : Outport
  TEMPSENS : Outport  Port=2
  TCO : Outport  Port=3
  OFF_T1 : Outport  Port=4
  TCS : Outport  Port=5
  SENS_T1 : Outport  Port=6
  wires:
  BUS I2C Read TCO/1 -> " 3"/1(In1)
  BUS I2C Read Tref/1 -> " 4"/1(In1)
  " "/1(Out1) -> Rate Transition3/1  "U1 CH3"
  Rate Transition3/1 -> SENS_T1/1
  BUS I2C Read TCS/1 -> " 2"/1(In1)
  BUS I2C Read OFF T1/1 -> " 1"/1(In1)
  BUS I2C Read TEMPSENS/1 -> " 5"/1(In1)
  BUS I2C Read SENS_T1/1 -> " "/1(In1)  "U1 CH3"
  " 1"/1(Out1) -> Rate Transition1/1
  " 2"/1(Out1) -> Rate Transition2/1
  " 3"/1(Out1) -> Rate Transition4/1
  " 4"/1(Out1) -> Rate Transition5/1
  " 5"/1(Out1) -> Rate Transition6/1
  Rate Transition1/1 -> OFF_T1/1
  Rate Transition2/1 -> TCS/1
  Rate Transition4/1 -> TCO/1
  Rate Transition6/1 -> TEMPSENS/1
  Rate Transition5/1 -> Tref/1

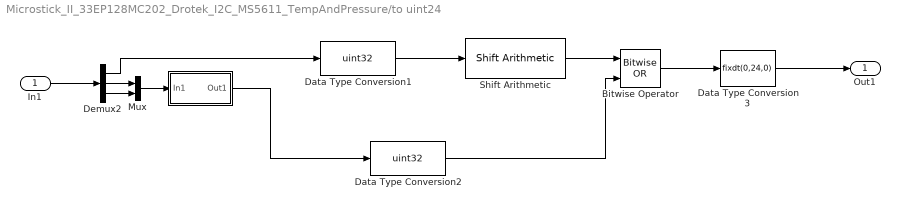
== system Microstick_II_33EP128MC202_Drotek_I2C_MS5611_TempAndPressure/to uint24 ==
  In1 : Inport
  " " : Subsystem
  Bitwise Operator : simulink/Logic and Bit Operations/Bitwise Operator  logicop=OR  UseBitMask=off  NumInputPorts=2  BitMask=bin2dec('11011001')  BitMaskRealWorld=Stored Integer
  Data Type Conversion1 : DataTypeConversion  OutDataTypeMode=uint32  OutDataTypeStr=uint32
  Data Type Conversion2 : DataTypeConversion  OutDataTypeMode=uint32  OutDataTypeStr=uint32
  Data Type Conversion3 : DataTypeConversion  OutDataTypeMode=Specify via dialog  OutDataType=fixdt(0,24,0)  OutDataTypeStr=fixdt(0,24,0)  ConvertRealWorld=Stored Integer (SI)
  Demux2 : Demux  Outputs=3
  Mux : Mux  Inputs=2
  Shift Arithmetic : simulink/Logic and Bit Operations/Shift Arithmetic  SystemSampleTime=-1  nBitShiftRight=-16  nBinPtShiftRight=0
  Out1 : Outport
  wires:
  In1/1 -> Demux2/1
  Shift Arithmetic/1 -> Bitwise Operator/1
  Demux2/1 -> Data Type Conversion1/1
  Mux/1 -> " "/1(In1)
  Demux2/2 -> Mux/1
  Bitwise Operator/1 -> Data Type Conversion3/1
  Demux2/3 -> Mux/2
  " "/1(Out1) -> Data Type Conversion2/1
  Data Type Conversion2/1 -> Bitwise Operator/2
  Data Type Conversion1/1 -> Shift Arithmetic/1
  Data Type Conversion3/1 -> Out1/1

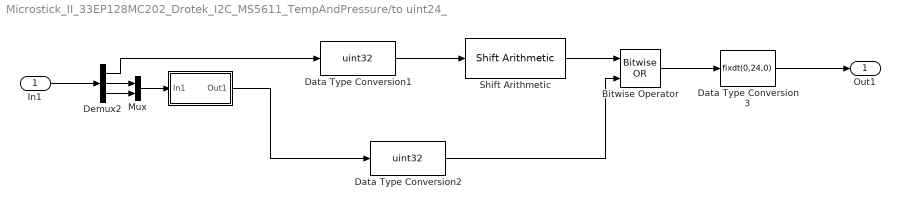
== system Microstick_II_33EP128MC202_Drotek_I2C_MS5611_TempAndPressure/to uint24_ ==
  In1 : Inport
  " " : Subsystem
  Bitwise Operator : simulink/Logic and Bit Operations/Bitwise Operator  logicop=OR  UseBitMask=off  NumInputPorts=2  BitMask=bin2dec('11011001')  BitMaskRealWorld=Stored Integer
  Data Type Conversion1 : DataTypeConversion  OutDataTypeMode=uint32  OutDataTypeStr=uint32
  Data Type Conversion2 : DataTypeConversion  OutDataTypeMode=uint32  OutDataTypeStr=uint32
  Data Type Conversion3 : DataTypeConversion  OutDataTypeMode=Specify via dialog  OutDataType=fixdt(0,24,0)  OutDataTypeStr=fixdt(0,24,0)  ConvertRealWorld=Stored Integer (SI)
  Demux2 : Demux  Outputs=3
  Mux : Mux  Inputs=2
  Shift Arithmetic : simulink/Logic and Bit Operations/Shift Arithmetic  SystemSampleTime=-1  nBitShiftRight=-16  nBinPtShiftRight=0
  Out1 : Outport
  wires:
  Data Type Conversion3/1 -> Out1/1
  Data Type Conversion1/1 -> Shift Arithmetic/1
  Data Type Conversion2/1 -> Bitwise Operator/2
  " "/1(Out1) -> Data Type Conversion2/1
  Demux2/3 -> Mux/2
  Bitwise Operator/1 -> Data Type Conversion3/1
  Demux2/2 -> Mux/1
  Mux/1 -> " "/1(In1)
  Demux2/1 -> Data Type Conversion1/1
  Shift Arithmetic/1 -> Bitwise Operator/1
  In1/1 -> Demux2/1

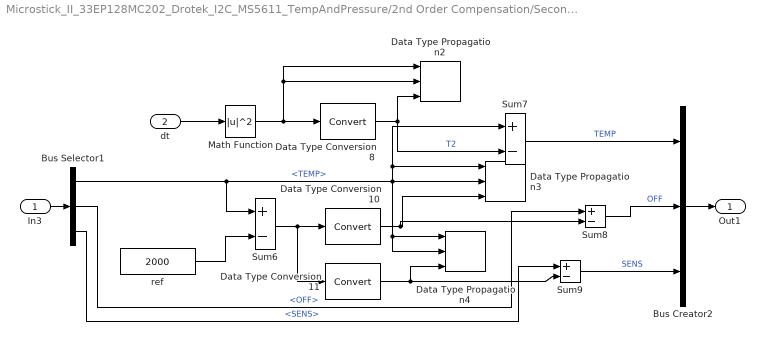
== system Microstick_II_33EP128MC202_Drotek_I2C_MS5611_TempAndPressure/2nd Order Compensation/Second Order Temp Compensation ==
  In3 : Inport
  dt : Inport  Port=2
  Bus Creator2 : BusCreator  Inputs=3
  Bus Selector1 : BusSelector  OutputSignals=TEMP,OFF,SENS
  Data Type Propagation2 : simulink/Signal Attributes/Data Type Propagation  PropDataType=fixdt(1, 16)  IfRefDouble=double  IfRefSingle=single  IsSigned=IsSigned1  NumBitsBase=NumBits1  NumBitsMult=1  NumBitsAdd=0  NumBitsAllowFinal=1:128  PropScaling=2^-10  ValuesUsedBestPrec=[5 -7]  SlopeBase=min([Slope1 Slope2])  SlopeMult=2^-31  SlopeAdd=0  BiasBase=Bias1  BiasMult=0  BiasAdd=0
  Data Type Propagation3 : simulink/Signal Attributes/Data Type Propagation  PropDataType=fixdt(1, 16)  IfRefDouble=double  IfRefSingle=single  IsSigned=IsSigned1  NumBitsBase=NumBits1  NumBitsMult=1  NumBitsAdd=0  NumBitsAllowFinal=1:128  PropScaling=2^-10  ValuesUsedBestPrec=[5 -7]  SlopeBase=Slope1  SlopeMult=5/2  SlopeAdd=0  BiasBase=Bias1  BiasMult=0  BiasAdd=0
  Data Type Propagation4 : simulink/Signal Attributes/Data Type Propagation  PropDataType=fixdt(1, 16)  IfRefDouble=double  IfRefSingle=single  IsSigned=IsSigned1  NumBitsBase=NumBits1  NumBitsMult=1  NumBitsAdd=0  NumBitsAllowFinal=1:128  PropScaling=2^-10  ValuesUsedBestPrec=[5 -7]  SlopeBase=Slope1  SlopeMult=5/4  SlopeAdd=0  BiasBase=Bias1  BiasMult=0  BiasAdd=0
  Data Type Conversion10 : DataTypeConversion  ConvertRealWorld=Stored Integer (SI)
  Data Type Conversion11 : DataTypeConversion  ConvertRealWorld=Stored Integer (SI)
  Data Type Conversion8 : DataTypeConversion  ConvertRealWorld=Stored Integer (SI)
  Math Function : Math  Operator=magnitude^2  OutDataTypeStr=Inherit: Inherit via back propagation  SaturateOnIntegerOverflow=on
  Sum{6..9} (4 alike) : Sum  Inputs=+-  OutDataTypeStr=Inherit: Same as accumulator
  ref : Constant  Value=2000  OutDataTypeMode=uint16  OutDataTypeStr=uint16
  Out1 : Outport
  wires:
  Bus Selector1/3 -> Sum9/1  "<SENS>"
  Sum8/1 -> Bus Creator2/2  "OFF"
  Bus Selector1/2 -> Sum8/1  "<OFF>"
  Sum7/1 -> Bus Creator2/1  "TEMP"
  Sum9/1 -> Bus Creator2/3  "SENS"
  Data Type Conversion11/1 -> Data Type Propagation4/3, Sum9/2
  ref/1 -> Sum6/2
  Bus Creator2/1 -> Out1/1
  Bus Selector1/1 -> Data Type Propagation3/1, Sum7/1, Data Type Propagation4/1, Data Type Propagation4/2, Data Type Propagation3/2, Sum6/1  "<TEMP>"
  Sum6/1 -> Data Type Conversion10/1, Data Type Conversion11/1
  In3/1 -> Bus Selector1/1
  Data Type Conversion8/1 -> Data Type Propagation2/3, Sum7/2  "T2"
  dt/1 -> Math Function/1
  Math Function/1 -> Data Type Conversion8/1, Data Type Propagation2/1, Data Type Propagation2/2
  Data Type Conversion10/1 -> Data Type Propagation3/3, Sum8/2

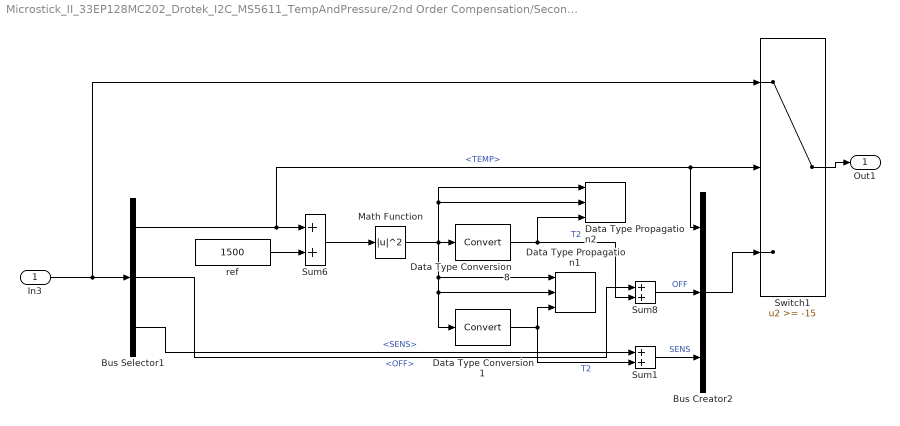
== system Microstick_II_33EP128MC202_Drotek_I2C_MS5611_TempAndPressure/2nd Order Compensation/Second Order Temp Compensation1 ==
  In3 : Inport
  Bus Creator2 : BusCreator  Inputs=3
  Bus Selector1 : BusSelector  OutputSignals=TEMP,OFF,SENS
  Data Type Propagation1 : simulink/Signal Attributes/Data Type Propagation  PropDataType=fixdt(1, 16)  IfRefDouble=double  IfRefSingle=single  IsSigned=IsSigned1  NumBitsBase=NumBits1  NumBitsMult=1  NumBitsAdd=0  NumBitsAllowFinal=1:128  PropScaling=2^-10  ValuesUsedBestPrec=[5 -7]  SlopeBase=min([Slope1 Slope2])  SlopeMult=11/2  SlopeAdd=0  BiasBase=Bias1  BiasMult=0  BiasAdd=0
  Data Type Propagation2 : simulink/Signal Attributes/Data Type Propagation  PropDataType=fixdt(1, 16)  IfRefDouble=double  IfRefSingle=single  IsSigned=IsSigned1  NumBitsBase=NumBits1  NumBitsMult=1  NumBitsAdd=0  NumBitsAllowFinal=1:128  PropScaling=2^-10  ValuesUsedBestPrec=[5 -7]  SlopeBase=min([Slope1 Slope2])  SlopeMult=7  SlopeAdd=0  BiasBase=Bias1  BiasMult=0  BiasAdd=0
  Data Type Conversion1 : DataTypeConversion  ConvertRealWorld=Stored Integer (SI)
  Data Type Conversion8 : DataTypeConversion  ConvertRealWorld=Stored Integer (SI)
  Math Function : Math  Operator=magnitude^2  OutDataTypeStr=Inherit: Inherit via back propagation  SaturateOnIntegerOverflow=on
  Sum1 : Sum  OutDataTypeStr=Inherit: Same as accumulator
  Sum6 : Sum  OutDataTypeStr=Inherit: Same as accumulator
  Sum8 : Sum  OutDataTypeStr=Inherit: Same as accumulator
  Switch1 : Switch  Threshold=-15  InputSameDT=on
  ref : Constant  Value=1500  OutDataTypeMode=uint16  OutDataTypeStr=uint16
  Out1 : Outport
  wires:
  In3/1 -> Switch1/1, Bus Selector1/1
  Sum8/1 -> Bus Creator2/2  "OFF"
  Bus Selector1/1 -> Switch1/2, Bus Creator2/1, Sum6/1  "<TEMP>"
  Math Function/1 -> Data Type Propagation1/1, Data Type Propagation1/2, Data Type Conversion1/1, Data Type Propagation2/2, Data Type Propagation2/1, Data Type Conversion8/1
  Data Type Conversion8/1 -> Sum8/2, Data Type Propagation2/3  "T2"
  Sum6/1 -> Math Function/1
  ref/1 -> Sum6/2
  Data Type Conversion1/1 -> Sum1/2, Data Type Propagation1/3  "T2"
  Sum1/1 -> Bus Creator2/3  "SENS"
  Bus Selector1/3 -> Sum1/1  "<SENS>"
  Bus Creator2/1 -> Switch1/3
  Switch1/1 -> Out1/1
  Bus Selector1/2 -> Sum8/1  "<OFF>"
